simulink model "observer"  (R2017b)
settings: Solver=ode45  StartTime=0.0  StopTime=1  RelTol=1e-3  EnableMultiTasking=on
values from neighbouring files (symbols this model uses):
  A = zeros(5,5)    [kalmanfilter.m]
  B = zeros(5,6)    [kalmanfilter.m]
  C = [ A(1:3,1:3), zeros(3,2); zeros(2,3), eye(2,2)]    [kalmanfilter.m]
  D = [ B(1:3,:) ; zeros(2,6) ]    [kalmanfilter.m]
undefined symbols (not defined in the file or in its folder): L
libraries: simulink x1
settings Model: Creator=nagamune  LastModifiedBy=Carter
settings DataIOCC: LimitDataPoints=on  SaveFormat=Array
settings OptimizationCC: LifeSpan=inf
settings DebuggingCC: SolverPrmCheckMsg=warning  SFUnexpectedBacktrackingDiag=warning  SFNoUnconditionalDefaultTransitionDiag=warning  SFExecutionAtInitializationDiag=none
settings HardwareCC: ProdBitPerPointer=32  ProdBitPerSizeT=32  ProdBitPerPtrDiffT=32  ProdLargestAtomicFloat=None  ProdIntDivRoundTo=Undefined  ProdEndianess=Unspecified  ProdWordSize=32  ProdHWDeviceType=32-bit Generic
settings ModelReferenceCC: PropagateSignalLabelsOutOfModel=off
settings CodeAppCC: StateflowObjectComments=on
settings GRTTargetCC: TargetLangStandard=C89/C90 (ANSI)  GeneratePreprocessorConditionals=Disable all
settings ConfigComp: CovMetricSettings=dw  CovHtmlReporting=on  CovSaveCumulativeToWorkspaceVar=on  CovSaveSingleToWorkspaceVar=on  CovExternalEMLEnable=off  CovSFcnEnable=off

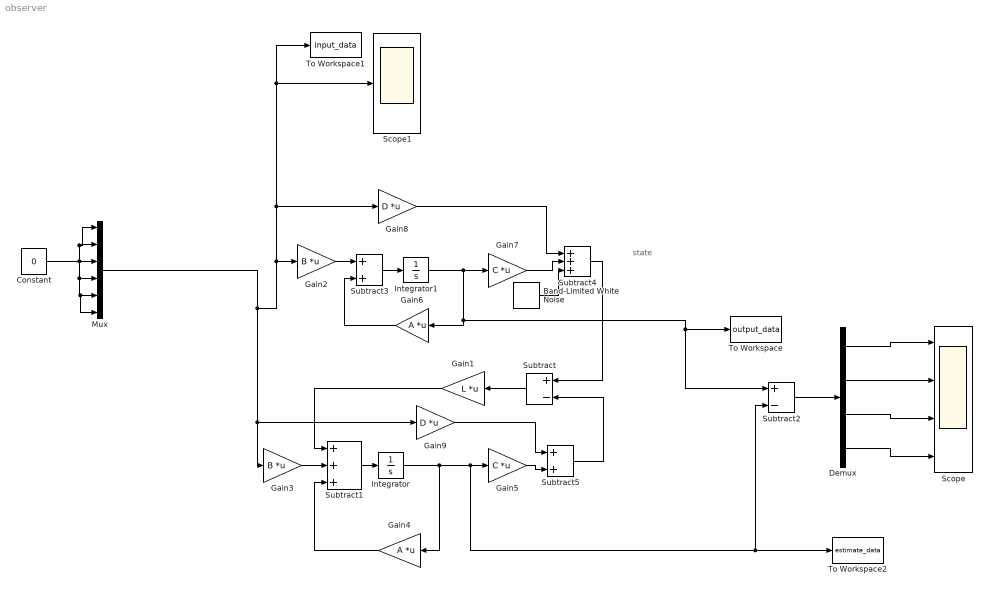
== system observer ==
  note: state
  Band-Limited White Noise : simulink/Sources/Band-Limited White Noise  Cov=[0.0025]  Ts=0.001  seed=[23341]
  Constant : Constant  Value=0
  Demux : Demux
  Gain1 : Gain  Gain=L  Multiplication=Matrix(K*u)
  Gain2 : Gain  Gain=B  Multiplication=Matrix(K*u)
  Gain3 : Gain  Gain=B  Multiplication=Matrix(K*u)
  Gain4 : Gain  Gain=A  Multiplication=Matrix(K*u)
  Gain5 : Gain  Gain=C  Multiplication=Matrix(K*u)
  Gain6 : Gain  Gain=A  Multiplication=Matrix(K*u)
  Gain7 : Gain  Gain=C  Multiplication=Matrix(K*u)
  Gain8 : Gain  Gain=D  Multiplication=Matrix(K*u)
  Gain9 : Gain  Gain=D  Multiplication=Matrix(K*u)
  Integrator : Integrator  InitialCondition=[0, 0, 0, 0, 0]
  Integrator1 : Integrator  InitialCondition=[0.1, 0.1, 0.1, 0, 0]
  Mux : Mux  Inputs=6
  Scope : Scope  NumInputPorts=4
  Scope1 : Scope
  Subtract : Sum  Inputs=+-
  Subtract1 : Sum  Inputs=+++
  Subtract2 : Sum  Inputs=+-
  Subtract3 : Sum
  Subtract4 : Sum  Inputs=+++
  Subtract5 : Sum
  To Workspace : ToWorkspace  VariableName=output_data  SaveFormat=Timeseries  SampleTime=-1
  To Workspace1 : ToWorkspace  VariableName=input_data  SaveFormat=Timeseries  SampleTime=-1
  To Workspace2 : ToWorkspace  VariableName=estimate_data  SaveFormat=Timeseries  SampleTime=-1
  wires:
  Subtract2/1 -> Demux/1
  Demux/1 -> Scope/1
  Demux/2 -> Scope/2
  Demux/3 -> Scope/3
  Demux/4 -> Scope/4
  Gain3/1 -> Subtract1/2
  Gain1/1 -> Subtract1/1
  Subtract/1 -> Gain1/1
  Gain4/1 -> Subtract1/3
  Mux/1 -> Gain9/1, Gain3/1, Gain8/1, To Workspace1/1, Scope1/1, Gain2/1
  Subtract1/1 -> Integrator/1
  Integrator/1 -> To Workspace2/1, Subtract2/2, Gain5/1, Gain4/1
  Constant/1 -> Mux/6, Mux/5, Mux/4, Mux/1, Mux/2, Mux/3
  Gain2/1 -> Subtract3/1
  Subtract3/1 -> Integrator1/1
  Gain6/1 -> Subtract3/2
  Integrator1/1 -> Gain7/1, To Workspace/1, Subtract2/1, Gain6/1
  Gain7/1 -> Subtract4/2
  Gain8/1 -> Subtract4/1
  Subtract4/1 -> Subtract/1
  Gain5/1 -> Subtract5/2
  Gain9/1 -> Subtract5/1
  Subtract5/1 -> Subtract/2
  Band-Limited White Noise/1 -> Subtract4/3
